simulink model "warteschlange_var2"  (Simulink 4.00)
settings: Solver=FixedStepDiscrete  StartTime=0.0  StopTime=500.0  RelTol=1e-3
settings Model: LastModifiedBy=Administrator  BlockReductionOpt=off

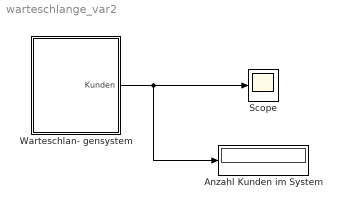
== system warteschlange_var2 ==
  Anzahl Kunden im System : Display
      settings: Format=short
  Scope : Scope
      settings: TimeRange=500  YMin=-1  YMax=1  SaveToWorkspace=off  SaveName=ScopeData  LimitDataPoints=on  MaxDataPoints=5000
  Warteschlan- gensystem : Stateflow chart
      settings: RTWFcnNameOpts=Auto  RTWFileNameOpts=Auto
  wires:
  Warteschlan- gensystem/1(Kunden) -> Scope/1, Anzahl Kunden im System/1

== stateflow chart Warteschlan- gensystem ==
  settings: updateMethod=DISCRETE  sampleTime=1  executeAtInitialization=1
  state Warteschlangensystem
    state Kunden_prozess/ [parallel]
      state Hilfszustand/
        entry:iz=imin+...
        (imax-imin)*...
        ml('rand');
        az=az+iz;
      (default) -> Hilfszustand
      Hilfszustand -> Hilfszustand : [t>=az]/Ankunft
    state Server_prozess/ [parallel]
      state idle/
      state busy/
        entry: sz=smin+(smax-smin)*ml('rand');
        bz=bz+sz;
        on Ankunft: Kunden=Kunden+1;
      (default) -> idle
      idle -> busy : Ankunft/Kunden=Kunden+1;bz=t;
      busy -> (junction 9) : [t>=bz]{Kunden=Kunden-1}
      (junction 9) -> idle : [Kunden==0]
      (junction 9) -> busy
  (default) -> Warteschlangensystem
  data: iz local int16; az local int16; sz local int16; Kunden output int16; bz local int16; smin constant double; smax constant double; imin local double; imax local double
  events: Ankunft local EITHER_EDGE_EVENT
